simulink model "sail_boat_simulator"  (R2017a)
settings: Solver=VariableStepAuto  StartTime=0.0  StopTime=5  RelTol=1e-3
libraries: fuzblock x1
settings Model: Creator=andre  LastModifiedBy=andre

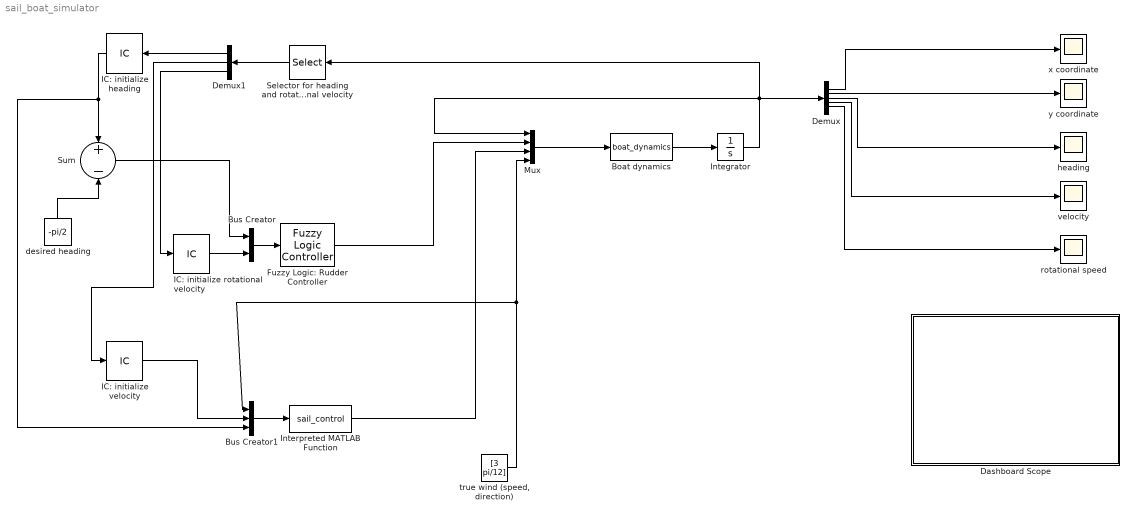
== system sail_boat_simulator ==
  Boat dynamics : MATLABFcn  MATLABFcn=boat_dynamics  OutputDimensions=5  Output1D=off
  Bus Creator : BusCreator  Inputs=2
  Bus Creator1 : BusCreator  Inputs=3
  Dashboard Scope : Subsystem  DialogController=hmiCreateDDGDialog  IsWebBlock=on  mask(MWDashboardBlock){webBlockId=2034cc10-1aec-4d69-bfd4-850be5add699, webBlockType=sdiscope, ShowInitialText=on, HMISrcModelName=sail_boat_simulator}
      mask prompts: webBlockId "WebBlock Id"; webBlockType "WebBlock Type"; HMISrcModelName "Source Model"
      mask help: SimulinkHMI:dialogs:HMIScopeDialogDesc
      mask Help: helpview([docroot '/mapfiles/simulink.map'], 'hmi_scope')
      mask Display:
      | if strcmp(get_param(bdroot(gcb),'BlockDiagramType'), 'library')
      |     image([(matlabroot) '/toolbox/simulink/hmi/icons/DashboardScope.png']);
      | end
  Demux : Demux  Outputs=5
  Demux1 : Demux  Outputs=3
  Fuzzy Logic: Rudder Controller : fuzblock/Fuzzy Logic  Controller  fis='rudder_control.fis'
  IC: initialize rotational velocity : InitialCondition  Value=0
  IC: initialize velocity : InitialCondition  Value=0
  IC: initialize heading : InitialCondition  Value=0
  Integrator : Integrator  InitialCondition=[0 0 pi/12 1 1]
  Interpreted MATLAB Function : MATLABFcn  MATLABFcn=sail_control
  Mux : Mux
  Selector for heading and rotational velocity : Selector  InputPortWidth=5  IndexOptions=Index vector (dialog)  Indices="[3  5]"  OutputSizes=1
  Sum : Sum  Inputs=+-
  desired heading : Constant  Value=-pi/2
  heading : Scope
  rotational speed : Scope
  "true wind (speed, direction)" : Constant  Value=[3 pi/12]  VectorParams1D=off
  velocity : Scope
  x coordinate : Scope
  y coordinate : Scope
  wires:
  Mux/1 -> Boat dynamics/1
  Boat dynamics/1 -> Integrator/1
  Integrator/1 -> Selector for heading and rotational velocity/1, Demux/1, Mux/1
  Demux/1 -> x coordinate/1
  Demux/2 -> y coordinate/1
  Demux/3 -> heading/1
  Demux/4 -> velocity/1
  Demux/5 -> rotational speed/1
  "true wind (speed, direction)"/1 -> Mux/4, Bus Creator1/1
  Fuzzy Logic: Rudder Controller/1 -> Mux/2
  Interpreted MATLAB Function/1 -> Mux/3
  desired heading/1 -> Sum/2
  Sum/1 -> Bus Creator/1
  Bus Creator/1 -> Fuzzy Logic: Rudder Controller/1
  Selector for heading and rotational velocity/1 -> Demux1/1
  IC: initialize heading/1 -> Bus Creator1/3, Sum/1
  Demux1/1 -> IC: initialize heading/1
  IC: initialize rotational velocity/1 -> Bus Creator/2
  Bus Creator1/1 -> Interpreted MATLAB Function/1
  Demux1/3 -> IC: initialize rotational velocity/1
  IC: initialize velocity/1 -> Bus Creator1/2
  Demux1/2 -> IC: initialize velocity/1

== system sail_boat_simulator/Dashboard Scope ==
